simulink model "ControlSystemExercise2"  (R2019b)
settings: Solver=VariableStepAuto  StartTime=0.0  StopTime=10.0  RelTol=1e-7  AbsTol=1e-7
libraries: simulink x1
settings Model: Creator=19398  LastModifiedBy=19398

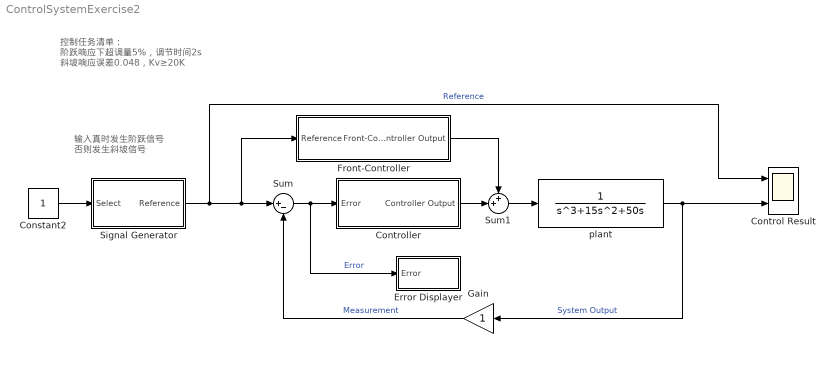
== system ControlSystemExercise2 ==
  note: 输入真时发生阶跃信号
      | 否则发生斜坡信号
  note: 控制任务清单：
      | 阶跃响应下超调量5%，调节时间2s
      | 斜坡响应误差0.048，Kv≥20K
  Constant2 : Constant
  Control Result : Scope  NumInputPorts=2
  Controller : Subsystem
  Error Displayer : Subsystem
  Front-Controller : Subsystem
  Gain : Gain
  Signal Generator : Subsystem
  Sum : Sum  Inputs=|+-
  Sum1 : Sum  Inputs=++|
  plant : TransferFcn  Denominator=[1 15 50 0]
  wires:
  plant/1 -> Control Result/2, Gain/1  "System Output"
  Sum/1 -> Error Displayer/1(Error), Controller/1(Error)  "Error"
  Controller/1(Controller Output) -> Sum1/2
  Sum1/1 -> plant/1
  Signal Generator/1(Reference) -> Control Result/1, Front-Controller/1(Reference), Sum/1  "Reference"
  Constant2/1 -> Signal Generator/1(Select)
  Front-Controller/1(Front-Controller Output) -> Sum1/1
  Gain/1 -> Sum/2  "Measurement"

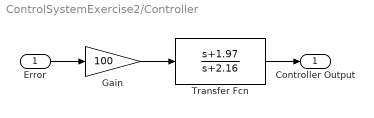
== system ControlSystemExercise2/Controller ==
  Error : Inport
  Gain : Gain  Gain=100
  Transfer Fcn : TransferFcn  Numerator=[1 1.97]  Denominator=[1 2.16]
  Controller Output : Outport
  wires:
  Gain/1 -> Transfer Fcn/1
  Error/1 -> Gain/1
  Transfer Fcn/1 -> Controller Output/1

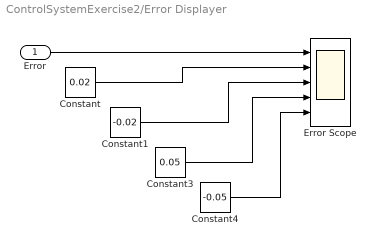
== system ControlSystemExercise2/Error Displayer ==
  Error : Inport
  Constant : Constant  Value=0.02
  Constant1 : Constant  Value=-0.02
  Constant3 : Constant  Value=0.05
  Constant4 : Constant  Value=-0.05
  Error Scope : Scope  NumInputPorts=5
  wires:
  Constant/1 -> Error Scope/2
  Constant3/1 -> Error Scope/4
  Constant1/1 -> Error Scope/3
  Error/1 -> Error Scope/1
  Constant4/1 -> Error Scope/5

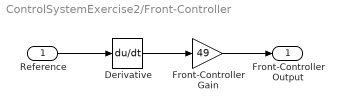
== system ControlSystemExercise2/Front-Controller ==
  Reference : Inport
  Derivative : Derivative  CoefficientInTFapproximation=10
  Front-Controller Gain : Gain  Gain=49
  Front-Controller Output : Outport
  wires:
  Reference/1 -> Derivative/1
  Derivative/1 -> Front-Controller Gain/1
  Front-Controller Gain/1 -> Front-Controller Output/1

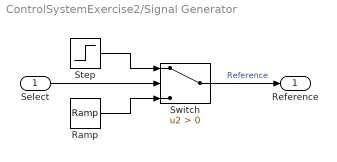
== system ControlSystemExercise2/Signal Generator ==
  Select : Inport
  Ramp : simulink/Sources/Ramp  slope=1  start=0  InitialOutput=0
  Step : Step  Time=0  SampleTime=0
  Switch : Switch  Criteria=u2 > Threshold
  Reference : Outport
  wires:
  Step/1 -> Switch/1
  Ramp/1 -> Switch/3
  Switch/1 -> Reference/1  "Reference"
  Select/1 -> Switch/2
